simulink model "arm_dynamics"  (R2016b)
settings: Solver=ode45  StartTime=0.0  StopTime=10.0  RelTol=1e-3  EnableMultiTasking=on
undefined symbols (not defined in the file): manipulator
libraries: roblocks x3
settings Model: Creator=zhonghang  LastModifiedBy=zhonghang
settings DataIOCC: LimitDataPoints=on  SaveFormat=Array
settings OptimizationCC: LifeSpan=inf
settings DebuggingCC: SFUnexpectedBacktrackingDiag=warning  SFNoUnconditionalDefaultTransitionDiag=warning  SFExecutionAtInitializationDiag=none
settings HardwareCC: ProdBitPerPointer=32  ProdBitPerSizeT=32  ProdBitPerPtrDiffT=32  ProdLargestAtomicFloat=None  ProdIntDivRoundTo=Undefined  ProdEndianess=Unspecified  ProdWordSize=32  ProdHWDeviceType=32-bit Generic
settings ModelReferenceCC: PropagateSignalLabelsOutOfModel=off
settings GRTTargetCC: TargetLangStandard=C89/C90 (ANSI)  GeneratePreprocessorConditionals=Disable all
settings ConfigComp: CovMetricSettings=dw  CovHtmlReporting=on  CovSaveCumulativeToWorkspaceVar=on  CovSaveSingleToWorkspaceVar=on  CovExternalEMLEnable=off

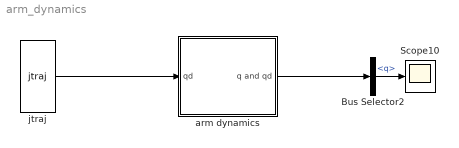
== system arm_dynamics ==
  Bus Selector2 : BusSelector  OutputSignals=q
  Scope10 : Scope
  arm dynamics : Subsystem  mask{robotarm=manipulator, q0=[-pi/3 3*pi/4 0 0]}
      mask prompts: robotarm "robot arm object"; q0 "joint initial value"
  jtraj : roblocks/Trajectory/jtraj  q0=[0 0 0 0]  qf=[pi pi/2 pi/2 0]  tmax=10  ts=-1
  wires:
  arm dynamics/1(q and qd) -> Bus Selector2/1
  jtraj/2 -> arm dynamics/1(qd)
  Bus Selector2/1 -> Scope10/1  "<q>"

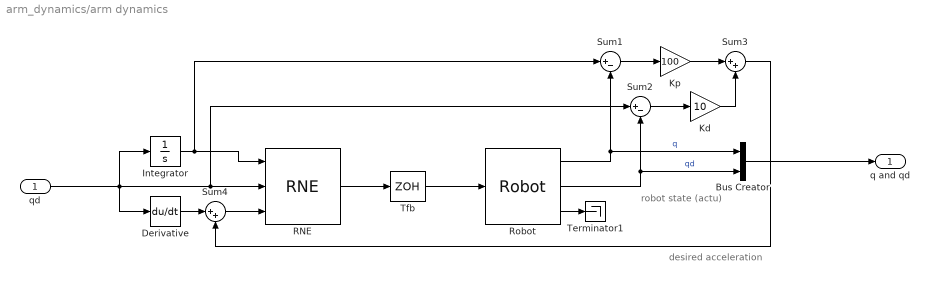
== system arm_dynamics/arm dynamics ==
  note: robot state
      | (actu)
  note: desired acceleration
  qd : Inport
  Bus Creator : BusCreator  Inputs=2
  Derivative : Derivative
  Integrator : Integrator
  Kd : Gain  Gain=10  SaturateOnIntegerOverflow=on  OutDataTypeStr=Inherit: Same as input  ParamDataTypeStr=Inherit: Same as input
  Kp : Gain  Gain=100  SaturateOnIntegerOverflow=on  OutDataTypeStr=Inherit: Same as input  ParamDataTypeStr=Inherit: Same as input
  RNE : roblocks/Dynamics/RNE  robot=robotarm  grav=[0 0 9.81]
  Robot : roblocks/Dynamics/Robot  robot=robotarm  q0=q0
  Sum1 : Sum  Inputs=|+-  SaturateOnIntegerOverflow=on  InputSameDT=on  OutDataTypeStr=Inherit: Same as first input
  Sum2 : Sum  Inputs=|+-  SaturateOnIntegerOverflow=on  InputSameDT=on  OutDataTypeStr=Inherit: Same as first input
  Sum3 : Sum  Inputs=|++  SaturateOnIntegerOverflow=on  InputSameDT=on  OutDataTypeStr=Inherit: Same as first input
  Sum4 : Sum  Inputs=|++  SaturateOnIntegerOverflow=on  InputSameDT=on  OutDataTypeStr=Inherit: Same as first input
  Terminator1 : Terminator
  Tfb : ZeroOrderHold  SampleTime=0.01
  q and qd : Outport
  wires:
  Tfb/1 -> Robot/1
  Sum4/1 -> RNE/3
  Robot/2 -> Bus Creator/2, Sum2/2  "qd"
  RNE/1 -> Tfb/1
  Robot/3 -> Terminator1/1
  Sum1/1 -> Kp/1
  Kp/1 -> Sum3/1
  Kd/1 -> Sum3/2
  qd/1 -> Integrator/1, Derivative/1, Sum2/1, RNE/2
  Robot/1 -> Bus Creator/1, Sum1/2  "q"
  Sum2/1 -> Kd/1
  Sum3/1 -> Sum4/2
  Bus Creator/1 -> q and qd/1
  Integrator/1 -> Sum1/1, RNE/1
  Derivative/1 -> Sum4/1
